simulink model "example_microCHP_modulating"  (R2016b)
settings: Solver=VariableStepAuto  StartTime=0.0  StopTime=10.0  RelTol=1e-3
libraries: carnot x2
settings Model: Creator=drhf  LastModifiedBy=drhf

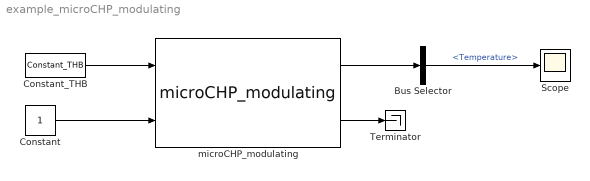
== system example_microCHP_modulating ==
  Bus Selector : BusSelector  OutputSignals=Temperature
  Constant : Constant
  Constant_THB : carnot/Source/Simple/Constant_THB  t=40  mdot=0  p=1e5  mID=No Pressure Drop  fluid=Water  mix=0  mix2=0  mix3=0  dia=0.02  hgt=0
  Scope : Scope
  Terminator : Terminator
  microCHP_modulating : carnot/Source/Cogeneration/microCHP_modulating  P_th_max=12500  P_th_min=3500  P_th_start=8000  f_P_el=0.37  T_flow_setpoint=80  T_flow_max=88  t_start=180  t_readjustment=450
  wires:
  Constant_THB/1 -> microCHP_modulating/1
  Constant/1 -> microCHP_modulating/2
  microCHP_modulating/1 -> Bus Selector/1
  Bus Selector/1 -> Scope/1  "<Temperature>"
  microCHP_modulating/2 -> Terminator/1
